simulink model "pendulum_sim"  (R2016b)
settings: Solver=ode45  StartTime=0.0  StopTime=P.t_end  RelTol=1e-3  EnableMultiTasking=on
InitFcn:
  | addpath ./..
  | pendulum_param
  | pendulumParamHWf
values from neighbouring files (symbols this model uses):
  K = 0.0075    [pendulumParamHWf.m]
undefined symbols (not defined in the file or in its folder): denC, numC, P, pendulum_animation
settings Model: Creator=beard  LastModifiedBy=mclain
settings DataIOCC: LimitDataPoints=on  SaveFormat=Array  SignalLoggingSaveFormat=ModelDataLogs
settings OptimizationCC: ExpressionDepthLimit=2147483647  InitFltsAndDblsToZero=on  LifeSpan=inf
settings DebuggingCC: UnderspecifiedInitializationDetection=Classic  MergeDetectMultiDrivingBlocksExec=none  SolverPrmCheckMsg=warning  FcnCallInpInsideContextMsg=warning  StateNameClashWarn=warning  SFUnexpectedBacktrackingDiag=warning  SFNoUnconditionalDefaultTransitionDiag=warning  SFExecutionAtInitializationDiag=none
settings HardwareCC: ProdBitPerPointer=32  ProdBitPerSizeT=32  ProdBitPerPtrDiffT=32  ProdLargestAtomicFloat=None  ProdIntDivRoundTo=Undefined  ProdEndianess=Unspecified  ProdWordSize=32  ProdHWDeviceType=32-bit Generic
settings ModelReferenceCC: PropagateSignalLabelsOutOfModel=off
settings GRTTargetCC: TargetLangStandard=C89/C90 (ANSI)  GeneratePreprocessorConditionals=Disable all  CombineOutputUpdateFcns=off  GRTInterface=on
settings ConfigComp: CovMetricSettings=dw  CovHtmlReporting=on  CovSaveCumulativeToWorkspaceVar=on  CovSaveSingleToWorkspaceVar=on  CovExternalEMLEnable=off

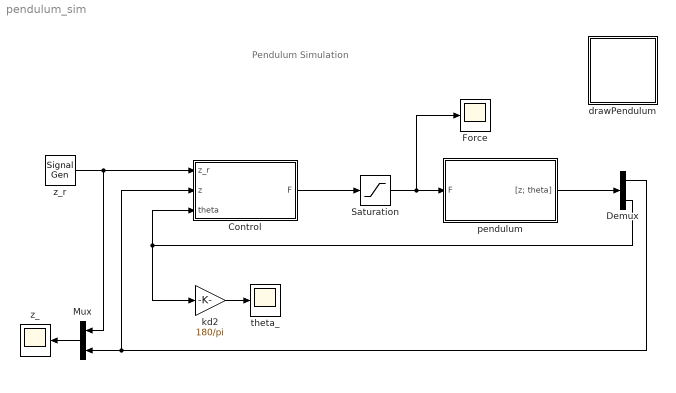
== system pendulum_sim ==
  note: Pendulum Simulation
  Control : Subsystem
  Demux : Demux  Outputs=2
  Force : Scope
  Mux : Mux  Inputs=2
  Saturation : Saturate  UpperLimit=P.F_max  LowerLimit=-P.F_max
  drawPendulum : Subsystem
      mask Display: image(imread('tv.jpg'))
  kd2 : Gain  Gain=180/pi
  pendulum : Subsystem
  theta_ : Scope
  z_ : Scope
  z_r : SignalGenerator  WaveForm=square  Amplitude=0.5  Frequency=.025
  wires:
  Saturation/1 -> pendulum/1(F), Force/1
  Control/1(F) -> Saturation/1
  pendulum/1("[z; theta]") -> Demux/1
  Demux/2 -> kd2/1, Control/3(theta)
  Demux/1 -> Control/2(z), Mux/2
  z_r/1 -> Mux/1, Control/1(z_r)
  Mux/1 -> z_/1
  kd2/1 -> theta_/1

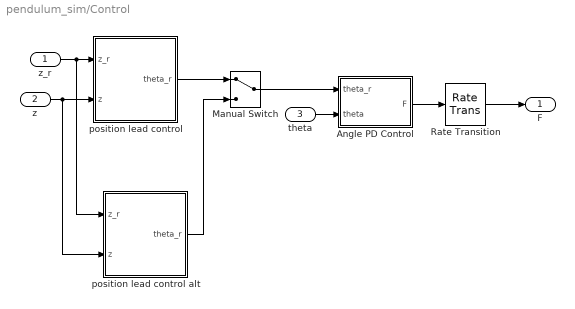
== system pendulum_sim/Control ==
  z_r : Inport
  z : Inport  Port=2
  theta : Inport  Port=3
  "Angle PD Control " : Subsystem
  Manual Switch : ManualSwitch
  Rate Transition : RateTransition  OutPortSampleTime=P.Ts
  position lead control : Subsystem
  position lead control alt : Subsystem
  F : Outport
  wires:
  theta/1 -> "Angle PD Control "/2(theta)
  z_r/1 -> position lead control alt/1(z_r), position lead control/1(z_r)
  "Angle PD Control "/1(F) -> Rate Transition/1
  z/1 -> position lead control alt/2(z), position lead control/2(z)
  Rate Transition/1 -> F/1
  position lead control alt/1(theta_r) -> Manual Switch/2
  position lead control/1(theta_r) -> Manual Switch/1
  Manual Switch/1 -> "Angle PD Control "/1(theta_r)

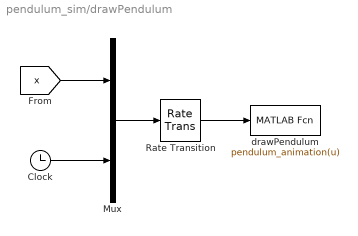
== system pendulum_sim/drawPendulum ==
  Clock : Clock
  Mux : Mux  Inputs=2
  Rate Transition : RateTransition  OutPortSampleTime=P.t_plot
  drawPendulum : MATLABFcn  MATLABFcn=pendulum_animation(u)  OutputDimensions=0
  wires:
  Mux/1 -> Rate Transition/1
  [x] -> Mux/1
  Clock/1 -> Mux/2
  Rate Transition/1 -> drawPendulum/1

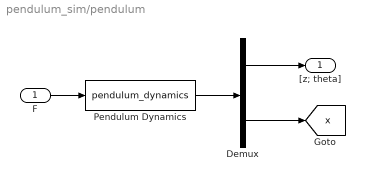
== system pendulum_sim/pendulum ==
  F : Inport
  Demux : Demux  Outputs=[2;4]
  Pendulum Dynamics : S-Function  FunctionName=pendulum_dynamics  Parameters=P  SFunctionDeploymentMode=off  EnableBusSupport=off
  "[z; theta]" : Outport
  tag scope: x=global
  wires:
  F/1 -> Pendulum Dynamics/1
  Pendulum Dynamics/1 -> Demux/1
  Demux/1 -> "[z; theta]"/1
  Demux/2 -> [x]

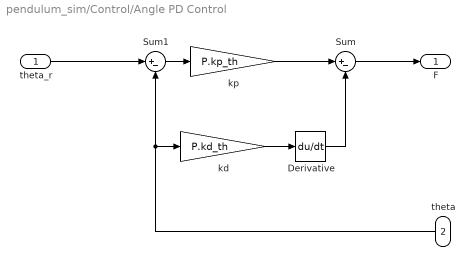
== system pendulum_sim/Control/Angle PD Control  ==
  theta_r : Inport
  theta : Inport  Port=2
  Derivative : Derivative  CoefficientInTFapproximation=P.sigma
  Sum : Sum  Inputs=|+-
  Sum1 : Sum  Inputs=|+-
  kd : Gain  Gain=P.kd_th
  kp : Gain  Gain=P.kp_th
  F : Outport
  wires:
  theta_r/1 -> Sum1/1
  Sum/1 -> F/1
  theta/1 -> kd/1, Sum1/2
  Sum1/1 -> kp/1
  kp/1 -> Sum/1
  kd/1 -> Derivative/1
  Derivative/1 -> Sum/2

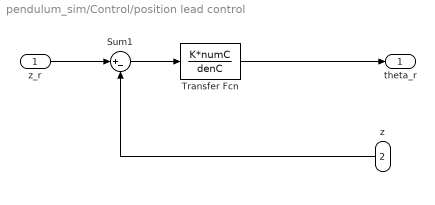
== system pendulum_sim/Control/position lead control ==
  z_r : Inport
  z : Inport  Port=2
  Sum1 : Sum  Inputs=|+-
  Transfer Fcn : TransferFcn  Numerator=K*numC  Denominator=denC
  theta_r : Outport
  wires:
  z_r/1 -> Sum1/1
  Sum1/1 -> Transfer Fcn/1
  Transfer Fcn/1 -> theta_r/1
  z/1 -> Sum1/2

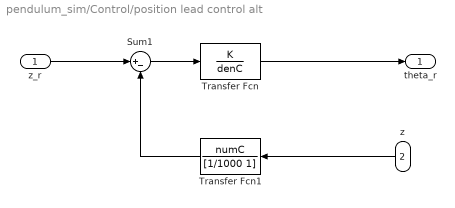
== system pendulum_sim/Control/position lead control alt ==
  z_r : Inport
  z : Inport  Port=2
  Sum1 : Sum  Inputs=|+-
  Transfer Fcn : TransferFcn  Numerator=K  Denominator=denC
  Transfer Fcn1 : TransferFcn  Numerator=numC  Denominator=[1/1000 1]
  theta_r : Outport
  wires:
  Sum1/1 -> Transfer Fcn/1
  Transfer Fcn/1 -> theta_r/1
  Transfer Fcn1/1 -> Sum1/2
  z/1 -> Transfer Fcn1/1
  z_r/1 -> Sum1/1
